simulink model "r2iq2xpfb14mcr17gb"  (R2012b)
settings: Solver=VariableStepDiscrete  SolverMode=SingleTasking  StartTime=0.0  StopTime=10.0  RelTol=1e-3
undefined symbols (not defined in the file or in its folder): pfb_coeff_gen_calc
libraries: xbsIndex_r4 x7879, casper_library_misc x39, casper_library_delays x20, xps_library x7
(part 8 of 95)

== system r2iq2xpfb14mcr17gb/fft/fft_direct ==
  sync : Inport
  shift : Inport  Port=2
  in00 : Inport  Port=3
  in01 : Inport  Port=4
  abus : Subsystem  AncestorBlock=casper_library_flow_control/bus_create  mask(bus_create){inputNum=1}
      mask prompts: inputNum "Number of inputs:"
      mask init:
      | bus_create_init(gcb,...
      |     'inputNum', inputNum);
  adebus0_0 : Subsystem  AncestorBlock=casper_library_flow_control/bus_expand  mask(bus_expand){mode=divisions of equal size, outputNum=1, outputWidth=36, outputBinaryPt=0, outputArithmeticType=0, show_format=off, outputToWorkspace=off, variablePrefix=out, outputToModelAsWell=on}
      mask prompts: outputNum "Number of outputs:"; outputWidth "Output width:"; outputBinaryPt "Output binary point position:"; outputArithmeticType "Output arithmetic type (ufix=0, fix=1, bool=2):"; show_format "Print format string?"; outputToWorkspace "Output to workspace?"; variablePrefix "Variable name prefix:"; outputToModelAsWell "Output to model as well?"
      mask help:
      | Expands a 'bus' made using a bus_create or Xilinx
      | concat block.
      | The input will be divided into the specified number
      | of outputs with the specified arithmetic types.
      | Divisions are made from most significant bit.
      mask init: same as r2iq2xpfb14mcr17gb/bus_expand1
      settings: AttributesFormatString=1 outputs
      mask TypeOptions mode: divisions of equal size | divisions of arbitrary size
      mask Callback mode: bus_expand_callback();
      mask Callback outputWidth: bus_expand_callback();
      mask Callback outputToWorkspace: bus_expand_callback();
  bbus : Subsystem  AncestorBlock=casper_library_flow_control/bus_create  mask(bus_create){inputNum=1}
      mask prompts: inputNum "Number of inputs:"
      mask init:
      | bus_create_init(gcb,...
      |     'inputNum', inputNum);
  bdebus0_0 : Subsystem  AncestorBlock=casper_library_flow_control/bus_expand  mask(bus_expand){mode=divisions of equal size, outputNum=1, outputWidth=36, outputBinaryPt=0, outputArithmeticType=0, show_format=off, outputToWorkspace=off, variablePrefix=out, outputToModelAsWell=on}
      mask prompts: outputNum "Number of outputs:"; outputWidth "Output width:"; outputBinaryPt "Output binary point position:"; outputArithmeticType "Output arithmetic type (ufix=0, fix=1, bool=2):"; show_format "Print format string?"; outputToWorkspace "Output to workspace?"; variablePrefix "Variable name prefix:"; outputToModelAsWell "Output to model as well?"
      mask help:
      | Expands a 'bus' made using a bus_create or Xilinx
      | concat block.
      | The input will be divided into the specified number
      | of outputs with the specified arithmetic types.
      | Divisions are made from most significant bit.
      mask init: same as r2iq2xpfb14mcr17gb/bus_expand1
      settings: AttributesFormatString=1 outputs
      mask TypeOptions mode: divisions of equal size | divisions of arbitrary size
      mask Callback mode: bus_expand_callback();
      mask Callback outputWidth: bus_expand_callback();
      mask Callback outputToWorkspace: bus_expand_callback();
  butterfly0_0 : Subsystem  AncestorBlock=casper_library_ffts/butterfly_direct  mask(butterfly_direct){n_inputs=1, biplex=off, FFTSize=14, Coeffs=[ 0 4096 2048 6144 1024 5120 3072 7168 512 4608 2560 6656 1536 5632 3584 7680 256 4352 2304 6400 1280 5376 3328 7424 768 4864 2816 6912 1792 5888 3840 7936 128 4224 2176 6272 1152 5248 3200 7296 640 4736 2688 6784 1664 5760 3712 7808 384 4480 2432 6528 1408 5504 3456 7552 896 4992 2944 7040 1920 6016 3968 8064 64 4160 2112 6208 1088 5184 3136 7232 576 4672 2624 6720 1600 5696 3648 7744 320 4416 2368 6464 1344 5440 3392 7488 832 4928 2880 6976 1856 5952 3904 8000 192 4288 2240 6336 1216 5312 3264 7360 704 4800 2752 6848 1728 5824 3776 7872 448 4544 2496 6592 1472 5568 3520 7616 960 5056 3008 7104 1984 6080 4032 8128 32 4128 2080 6176 1056 5152 3104 7200 544 4640 2592 6688 1568 5664 3616 7712 288 4384 2336 6432 1312 5408 3360 7456 800 4896 2848 6944 1824 5920 3872 7968 160 4256 2208 6304 1184 5280 3232 7328 672 4768 2720 6816 1696 5792 3744 7840 416 4512 2464 6560 1440 5536 3488 7584 928 5024 2976 7072 1952 6048 4000 8096 96 4192 2144 6240 1120 5216 3168 7264 608 4704 2656 6752 1632 5728 3680 7776 352 4448 2400 6496 1376 5472 3424 7520 864 4960 2912 7008 1888 5984 3936 8032 224 4320 2272 6368 1248 5344 3296 7392 736 4832 2784 6880 1760 5856 3808 7904 480 4576 2528 6624 1504 5600 3552 7648 992 5088 3040 7136 2016 6112 4064 8160 16 4112 2064 6160 1040 5136 3088 7184 528 4624 2576 6672 1552 5648 3600 7696 272 4368 2320 6416 1296 5392 3344 7440 784 4880 2832 6928 1808 5904 3856 7952 144 4240 2192 6288 1168 5264 3216 7312 656 4752 2704 6800 1680 5776 3728 7824 400 4496 2448 6544 1424 5520 3472 7568 912 5008 2960 7056 1936 6032 3984 8080 80 4176 2128 6224 1104 5200 3152 7248 592 4688 2640 6736 1616 5712 3664 7760 336 4432 2384 6480 1360 5456 3408 7504 848 4944 2896 6992 1872 5968 3920 8016 208 4304 2256 6352 1232 5328 3280 7376 720 4816 2768 6864 1744 5840 3792 7888 464 4560 2512 6608 1488 5584 3536 7632 976 5072 3024 7120 2000 6096 4048 8144 48 4144 2096 6192 1072 5168 3120 7216 560 4656 2608 6704 1584 5680 3632 7728 304 4400 2352 6448 1328 5424 3376 7472 816 4912 2864 6960 1840 5936 3888 7984 176 4272 2224 6320 1200 5296 3248 7344 688 4784 2736 6832 1712 5808 3760 7856 432 4528 2480 6576 1456 5552 3504 7600 944 5040 2992 7088 1968 6064 4016 8112 112 4208 2160 6256 1136 5232 3184 7280 624 4720 2672 6768 1648 5744 3696 7792 368 4464 2416 6512 1392 5488 3440 7536 880 4976 2928 7024 1904 6000 3952 8048 240 4336 2288 6384 1264 5360 3312 7408 752 4848 2800 6896 1776 5872 3824 7920 496 4592 2544 6640 1520 5616 3568 7664 1008 5104 3056 7152 2032 6128 4080 8176 8 4104 2056 6152 1032 5128 3080 7176 520 4616 2568 6664 1544 5640 3592 7688 264 4360 2312 6408 1288 5384 3336 7432 776 4872 2824 6920 1800 5896 3848 7944 136 4232 2184 6280 1160 5256 3208 7304 648 4744 2696 6792 1672 5768 3720 7816 392 4488 2440 6536 1416 5512 3464 7560 904 5000 2952 7048 1928 6024 3976 8072 72 4168 2120 6216 1096 5192 3144 7240 584 4680 2632 6728 1608 5704 3656 7752 328 4424 2376 6472 1352 5448 3400 7496 840 4936 2888 6984 1864 5960 3912 8008 200 4296 2248 6344 1224 5320 3272 7368 712 4808 2760 6856 1736 5832 3784 7880 456 4552 2504 6600 1480 5576 3528 7624 968 5064 3016 7112 1992 6088 4040 8136 40 4136 2088 6184 1064 5160 3112 7208 552 4648 2600 6696 1576 5672 3624 7720 296 4392 2344 6440 1320 5416 3368 7464 808 4904 2856 6952 1832 5928 3880 7976 168 4264 2216 6312 1192 5288 3240 7336 680 4776 2728 6824 1704 5800 3752 7848 424 4520 2472 6568 1448 5544 3496 7592 936 5032 2984 7080 1960 6056 4008 8104 104 4200 2152 6248 1128 5224 3176 7272 616 4712 2664 6760 1640 5736 3688 7784 360 4456 2408 6504 1384 5480 3432 7528 872 4968 2920 7016 1896 5992 3944 8040 232 4328 2280 6376 1256 5352 3304 7400 744 4840 2792 6888 1768 5864 3816 7912 488 4584 2536 6632 1512 5608 3560 7656 1000 5096 3048 7144 2024 6120 4072 8168 24 4120 2072 6168 1048 5144 3096 7192 536 4632 2584 6680 1560 5656 3608 7704 280 4376 2328 6424 1304 5400 3352 7448 792 4888 2840 6936 1816 5912 3864 7960 152 4248 2200 6296 1176 5272 3224 7320 664 4760 2712 6808 1688 5784 3736 7832 408 4504 2456 6552 1432 5528 ...(+35854 chars)], StepPeriod=0, coeff_bit_width=18, input_bit_width=18, bin_pt_in=17, downshift=off, async=off, add_latency=2, mult_latency=2, bram_latency=2, conv_latency=1, quantization=Round  (unbiased: +/- Inf), overflow=Saturate, coeffs_bit_limit=8, coeff_sharing=on, coeff_decimation=on, coeff_generation=on, cal_bits=1, n_bits_rotation=25, max_fanout=4, use_hdl=on, use_embedded=off, bitgrowth=off, hardcode_shifts=off, dsp48_adders=on}
      mask prompts: n_inputs "number inputs"; biplex "Used in biplex FFT"; FFTSize "Size of FFT: (2^? pts)"; Coeffs "Coefficients: (0 to 2^(FFTSize-1)-1)"; StepPeriod "Coefficient Step Period: (2^?)"; coeff_bit_width "Coefficient Bit Width"; input_bit_width "Input Bit Width"; bin_pt_in "Input binary point"; async "asynchronous operation"; add_latency "Add Latency"; mult_latency "Mult Latency"; bram_latency "BRAM Latency"; conv_latency "Convert latency"; quantization "Quantization Behavior"; overflow "Overflow Behavior"; coeffs_bit_limit "Number bits above which to store stage's coefficients in BRAM (2^? bits)"; coeff_sharing "BRAM sharing in coeff storage"; coeff_decimation "Store a fraction of coeff factors where useful"; coeff_generation "Generate coeffs with multipliers where useful"; cal_bits "Number calibration locations when generating coeffs (2^?)"; n_bits_rotation "Feedback rotation vector resolution"; max_fanout "Maximum fanout"; use_hdl "Use behavioural HDL for multipliers"; use_embedded "Use embedded multipliers"; bitgrowth "Bit growth instead of shifting"; hardcode_shifts "Hardcode shift schedule"; dsp48_adders "Use DSP48s for adders"
      mask help: FFT internal block.
      mask init:
      | butterfly_direct_init(gcb, ...
      |    'n_inputs', n_inputs, ...
      |    'biplex', biplex, ...
      |    'FFTSize', FFTSize, ...
      |    'Coeffs', Coeffs, ...
      |    'StepPeriod', StepPeriod, ...
      |    'coeff_bit_width', coeff_bit_width, ...
      |    'input_bit_width', input_bit_width, ...
      |    'bin_pt_in', bin_pt_in, ...
      |    'hardcode_shifts', hardcode_shifts, ...
      |    'bitgrowth', bitgrowth, ...
      |    'downshift', downshift, ...
      |    'async', async, ...
      |    'add_latency', add_latency, ...
      |    'mult_latency', mult_latency, ...
      |    'bram_latency', bram_latency, ...
      |    'conv_latency', conv_latency, ...
      |    'quantization', quantization, ...
      |    'overflow', overflow, ...
      |    'coeffs_bit_limit', coeffs_bit_limit, ...    
      |    'coeff_sharing', coeff_sharing, ...
      |    'coeff_decimation', coeff_decimation, ...
      |    'coeff_generation', coeff_generation, ...
      |    'cal_bits', cal_bits, ...
      |    'n_bits_rotation', n_bits_rotation, ...
      |    'max_fanout', max_fanout, ...
      |    'use_hdl', use_hdl, ...
      |    'use_embedded', use_embedded, ...
      |    'dsp48_adders', dsp48_adders);
      settings: AttributesFormatString=twiddle_general
      mask TypeOptions quantization: Truncate | Round  (unbiased: +/- Inf) | Round  (unbiased: Even Values)
      mask TypeOptions overflow: Wrap | Saturate | Error
      mask Callback use_hdl:
      | % make mutually exclusive with use_embedded.
      | 
      | use_hdl = get_param(gcb, 'use_hdl');
      | if strcmp(use_hdl, 'on'),
      |     set_param_state(gcb, 'use_embedded', 'off');
      | else
      |     set_param_state(gcb, 'use_embedded', 'on');
      | end
      mask Callback use_embedded:
      | % make mutually exclusive with use_hdl.
      | 
      | use_hdl = get_param(gcb, 'use_embedded');
      | if strcmp(use_hdl, 'on'),
      |     set_param_state(gcb, 'use_hdl', 'off');
      | else
      |     set_param_state(gcb, 'use_hdl', 'on');
      | end
      mask Callback hardcode_shifts:
      | hardcode_shifts = get_param(gcb, 'hardcode_shifts');
      | set_param_state(gcb, 'downshift', hardcode_shifts);
      mask Callback dsp48_adders: %fft_callback_dsp48_adders(gcb);
  slice0 : xbsIndex_r4/Slice  nbits=1  boolean_output=on  mode=Lower Bit Location + Width  bit1=0  base1=MSB of Input  bit0=0  base0=LSB of Input  dbl_ovrd=off  block_type=slice
  sync_out : Outport
  out00 : Outport  Port=2
  out01 : Outport  Port=3
  of : Outport  Port=4
  wires:
  in00/1 -> abus/1(in1)
  adebus0_0/1(msb_lsb_out1) -> out00/1
  in01/1 -> bbus/1(in1)
  bdebus0_0/1(msb_lsb_out1) -> out01/1
  shift/1 -> slice0/1
  sync/1 -> butterfly0_0/3(sync_in)
  butterfly0_0/4(sync_out) -> sync_out/1
  slice0/1 -> butterfly0_0/4(shift)
  abus/1(bus_out) -> butterfly0_0/1(a)
  bbus/1(bus_out) -> butterfly0_0/2(b)
  butterfly0_0/3(of) -> of/1
  butterfly0_0/1(a+bw) -> adebus0_0/1(bus_in)
  butterfly0_0/2(a-bw) -> bdebus0_0/1(bus_in)
